simulink model "five_bar_model"  (R2018a)
settings: Solver=ode4  StartTime=0.0  StopTime=10  FixedStep=0.0001  RelTol=1e-3
values from neighbouring files (symbols this model uses):
  g = 9.80665    [ddyn5.m]    (also in idyn5.m = -9.80665; test_dynamics.m = -9.80665; test_model.m)
  q = [NaN; NaN; NaN; NaN; NaN]    [fkine5.m]    (also in ikine5.m = [q11;q12;q13;q21;q22])
  qa = [q11;q21]    [ikine5.m]    (also in model_parameters_v_1.m = ones(length(q_(1,:)),1) * 50; test_model.m = [q(1,:);q(4,:)])
  t0r = J * qda    [ffirstkine5.m]    (also in test_dynamics.m = [0;0]; test_kinematics.m = [1;1]; test_model.m = p)
  t0rd = (J * qdda+ at)    [fsecondkine5.m]    (also in test_dynamics.m = [0;0]; test_kinematics.m = [-1;1]; test_model.m = p)
  x0 = p(1,1)    [model_parameters_v_1.m]    (also in test_model.m)
  y0 = p(2,1)    [model_parameters_v_1.m]    (also in test_model.m = p(1,2))
undefined symbols (not defined in the file or in its folder): X, Y, Z
libraries: sm_lib x23, simulink x10, nesl_utility x9, fl_lib x2
(part 1 of 2)
settings Model: Creator=jere  LastModifiedBy=jere

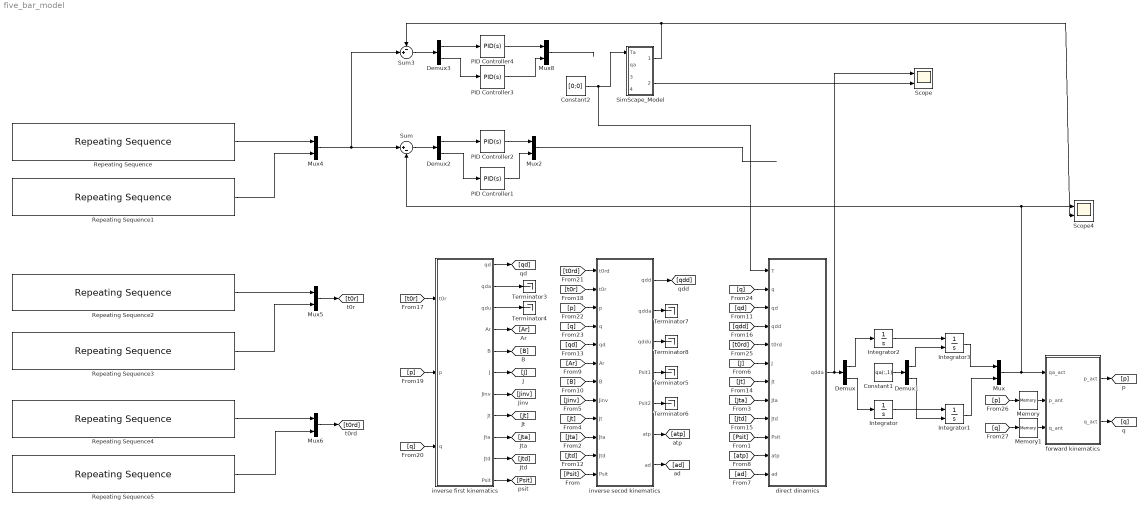
== system five_bar_model ==
  Constant1 : Constant  Value=qa(:,1)
  Constant2 : Constant  Value=[0;0]
  Demux{,1..3} (4 alike) : Demux  Outputs=2
  Integrator : Integrator
  Integrator1 : Integrator  InitialConditionSource=external  InitialCondition=0.3
  Integrator2 : Integrator
  Integrator3 : Integrator  InitialConditionSource=external
  Memory : Memory  InitialCondition=[x0;y0]  LinearizeAsDelay=on
  Memory1 : Memory  InitialCondition=q(:,1)  LinearizeAsDelay=on
  Mux{,2,4..6,8} (6 alike) : Mux  Inputs=2
  PID Controller1 : simulink/Continuous/PID Controller  Controller=PID  TimeDomain=Continuous-time  SampleTime=-1  IntegratorMethod=Forward Euler  FilterMethod=Forward Euler  Form=Parallel  UseFilter=on  ControllerParametersSource=internal  P=75.814948562535  I=487.355305210332  D=2.89544597191695  N=752.857471853223  InitialConditionSource=internal  InitialConditionForIntegrator=0  InitialConditionForFilter=0  ExternalReset=none  LimitOutput=off  UpperSaturationLimit=inf  LowerSaturationLimit=-inf  LinearizeAsGain=on  AntiWindupMode=none  Kb=1  TrackingMode=off  Kt=1  PParamMin=[]  PParamMax=[]  IParamMin=[]  IParamMax=[]  DParamMin=[]  DParamMax=[]  NParamMin=[]  NParamMax=[]  KbParamMin=[]  KbParamMax=[]  KtParamMin=[]  KtParamMax=[]  POutMin=[]  POutMax=[]  IOutMin=[]  IOutMax=[]  DOutMin=[]  DOutMax=[]  NOutMin=[]  NOutMax=[]  KbOutMin=[]  KbOutMax=[]  KtOutMin=[]  KtOutMax=[]  IntegratorOutMin=[]  IntegratorOutMax=[]  FilterOutMin=[]  FilterOutMax=[]  SumOutMin=[]  SumOutMax=[]  SumI1OutMin=[]  SumI1OutMax=[]  SumI2OutMin=[]  SumI2OutMax=[]  SumI3OutMin=[]  SumI3OutMax=[]  SumDOutMin=[]  SumDOutMax=[]  SaturationOutMin=[]  SaturationOutMax=[]  IntegratorContinuousStateAttributes=''  IntegratorStateMustResolveToSignalObject=off  IntegratorRTWStateStorageClass=Auto  FilterContinuousStateAttributes=''  FilterStateMustResolveToSignalObject=off  FilterRTWStateStorageClass=Auto  DifferentiatorICPrevScaledInput=0  DifferentiatorOutMin=[]  DifferentiatorOutMax=[]  FilterDiffOutCoefMin=[]  FilterDiffOutCoefMax=[]  SumDenOutMin=[]  SumDenOutMax=[]  SumNumOutMin=[]  SumNumOutMax=[]  ReciprocalOutMin=[]  ReciprocalOutMax=[]  DivideOutMin=[]  DivideOutMax=[]  TunerSelectOption=Transfer Function Based (PID Tuner App)
  PID Controller2 : simulink/Continuous/PID Controller  Controller=PID  TimeDomain=Continuous-time  SampleTime=-1  IntegratorMethod=Forward Euler  FilterMethod=Forward Euler  Form=Parallel  UseFilter=on  ControllerParametersSource=internal  P=103.663662761202  I=690.778716841285  D=2.91858268707005  N=267.25895733266  InitialConditionSource=internal  InitialConditionForIntegrator=0  InitialConditionForFilter=0  ExternalReset=none  LimitOutput=off  UpperSaturationLimit=inf  LowerSaturationLimit=-inf  LinearizeAsGain=on  AntiWindupMode=none  Kb=1  TrackingMode=off  Kt=1  PParamMin=[]  PParamMax=[]  IParamMin=[]  IParamMax=[]  DParamMin=[]  DParamMax=[]  NParamMin=[]  NParamMax=[]  KbParamMin=[]  KbParamMax=[]  KtParamMin=[]  KtParamMax=[]  POutMin=[]  POutMax=[]  IOutMin=[]  IOutMax=[]  DOutMin=[]  DOutMax=[]  NOutMin=[]  NOutMax=[]  KbOutMin=[]  KbOutMax=[]  KtOutMin=[]  KtOutMax=[]  IntegratorOutMin=[]  IntegratorOutMax=[]  FilterOutMin=[]  FilterOutMax=[]  SumOutMin=[]  SumOutMax=[]  SumI1OutMin=[]  SumI1OutMax=[]  SumI2OutMin=[]  SumI2OutMax=[]  SumI3OutMin=[]  SumI3OutMax=[]  SumDOutMin=[]  SumDOutMax=[]  SaturationOutMin=[]  SaturationOutMax=[]  IntegratorContinuousStateAttributes=''  IntegratorStateMustResolveToSignalObject=off  IntegratorRTWStateStorageClass=Auto  FilterContinuousStateAttributes=''  FilterStateMustResolveToSignalObject=off  FilterRTWStateStorageClass=Auto  DifferentiatorICPrevScaledInput=0  DifferentiatorOutMin=[]  DifferentiatorOutMax=[]  FilterDiffOutCoefMin=[]  FilterDiffOutCoefMax=[]  SumDenOutMin=[]  SumDenOutMax=[]  SumNumOutMin=[]  SumNumOutMax=[]  ReciprocalOutMin=[]  ReciprocalOutMax=[]  DivideOutMin=[]  DivideOutMax=[]  TunerSelectOption=Transfer Function Based (PID Tuner App)
  PID Controller3 : simulink/Continuous/PID Controller  Controller=PID  TimeDomain=Continuous-time  SampleTime=-1  IntegratorMethod=Forward Euler  FilterMethod=Forward Euler  Form=Parallel  UseFilter=on  ControllerParametersSource=internal  P=20220.2005625298  I=4298019.75181635  D=23.0115612854985  N=21654.4579542696  InitialConditionSource=internal  InitialConditionForIntegrator=0  InitialConditionForFilter=0  ExternalReset=none  LimitOutput=off  UpperSaturationLimit=inf  LowerSaturationLimit=-inf  LinearizeAsGain=on  AntiWindupMode=none  Kb=1  TrackingMode=off  Kt=1  PParamMin=[]  PParamMax=[]  IParamMin=[]  IParamMax=[]  DParamMin=[]  DParamMax=[]  NParamMin=[]  NParamMax=[]  KbParamMin=[]  KbParamMax=[]  KtParamMin=[]  KtParamMax=[]  POutMin=[]  POutMax=[]  IOutMin=[]  IOutMax=[]  DOutMin=[]  DOutMax=[]  NOutMin=[]  NOutMax=[]  KbOutMin=[]  KbOutMax=[]  KtOutMin=[]  KtOutMax=[]  IntegratorOutMin=[]  IntegratorOutMax=[]  FilterOutMin=[]  FilterOutMax=[]  SumOutMin=[]  SumOutMax=[]  SumI1OutMin=[]  SumI1OutMax=[]  SumI2OutMin=[]  SumI2OutMax=[]  SumI3OutMin=[]  SumI3OutMax=[]  SumDOutMin=[]  SumDOutMax=[]  SaturationOutMin=[]  SaturationOutMax=[]  IntegratorContinuousStateAttributes=''  IntegratorStateMustResolveToSignalObject=off  IntegratorRTWStateStorageClass=Auto  FilterContinuousStateAttributes=''  FilterStateMustResolveToSignalObject=off  FilterRTWStateStorageClass=Auto  DifferentiatorICPrevScaledInput=0  DifferentiatorOutMin=[]  DifferentiatorOutMax=[]  FilterDiffOutCoefMin=[]  FilterDiffOutCoefMax=[]  SumDenOutMin=[]  SumDenOutMax=[]  SumNumOutMin=[]  SumNumOutMax=[]  ReciprocalOutMin=[]  ReciprocalOutMax=[]  DivideOutMin=[]  DivideOutMax=[]  TunerSelectOption=Transfer Function Based (PID Tuner App)
  PID Controller4 : simulink/Continuous/PID Controller  Controller=PID  TimeDomain=Continuous-time  SampleTime=-1  IntegratorMethod=Forward Euler  FilterMethod=Forward Euler  Form=Parallel  UseFilter=on  ControllerParametersSource=internal  P=130671.244254794  I=70606761.3892061  D=48.6694021998481  N=21806.6233739507  InitialConditionSource=internal  InitialConditionForIntegrator=0  InitialConditionForFilter=0  ExternalReset=none  LimitOutput=off  UpperSaturationLimit=inf  LowerSaturationLimit=-inf  LinearizeAsGain=on  AntiWindupMode=none  Kb=1  TrackingMode=off  Kt=1  PParamMin=[]  PParamMax=[]  IParamMin=[]  IParamMax=[]  DParamMin=[]  DParamMax=[]  NParamMin=[]  NParamMax=[]  KbParamMin=[]  KbParamMax=[]  KtParamMin=[]  KtParamMax=[]  POutMin=[]  POutMax=[]  IOutMin=[]  IOutMax=[]  DOutMin=[]  DOutMax=[]  NOutMin=[]  NOutMax=[]  KbOutMin=[]  KbOutMax=[]  KtOutMin=[]  KtOutMax=[]  IntegratorOutMin=[]  IntegratorOutMax=[]  FilterOutMin=[]  FilterOutMax=[]  SumOutMin=[]  SumOutMax=[]  SumI1OutMin=[]  SumI1OutMax=[]  SumI2OutMin=[]  SumI2OutMax=[]  SumI3OutMin=[]  SumI3OutMax=[]  SumDOutMin=[]  SumDOutMax=[]  SaturationOutMin=[]  SaturationOutMax=[]  IntegratorContinuousStateAttributes=''  IntegratorStateMustResolveToSignalObject=off  IntegratorRTWStateStorageClass=Auto  FilterContinuousStateAttributes=''  FilterStateMustResolveToSignalObject=off  FilterRTWStateStorageClass=Auto  DifferentiatorICPrevScaledInput=0  DifferentiatorOutMin=[]  DifferentiatorOutMax=[]  FilterDiffOutCoefMin=[]  FilterDiffOutCoefMax=[]  SumDenOutMin=[]  SumDenOutMax=[]  SumNumOutMin=[]  SumNumOutMax=[]  ReciprocalOutMin=[]  ReciprocalOutMax=[]  DivideOutMin=[]  DivideOutMax=[]  TunerSelectOption=Transfer Function Based (PID Tuner App)
  Repeating Sequence : simulink/Sources/Repeating Sequence  rep_seq_t=0:10/49:10  rep_seq_y=qa(1,:)
  Repeating Sequence1 : simulink/Sources/Repeating Sequence  rep_seq_t=0:10/49:10  rep_seq_y=qa(2,:)
  Repeating Sequence2 : simulink/Sources/Repeating Sequence  rep_seq_t=0:10/49:10  rep_seq_y=t0r(:,1)'
  Repeating Sequence3 : simulink/Sources/Repeating Sequence  rep_seq_t=0:10/49:10  rep_seq_y=t0r(:,1)'
  Repeating Sequence4 : simulink/Sources/Repeating Sequence  rep_seq_t=0:10/49:10  rep_seq_y=t0rd(:,1)'
  Repeating Sequence5 : simulink/Sources/Repeating Sequence  rep_seq_t=0:10/49:10  rep_seq_y=t0rd(:,2)'
  Scope : Scope  NumInputPorts=2
  Scope4 : Scope  NumInputPorts=2
  SimScape_Model : Subsystem
  Sum : Sum  Inputs=|+-
  Sum3 : Sum  Inputs=-+|
  Terminator{3..8} (6 alike) : Terminator
  direct dinamics : MATLAB Function  TreatAsAtomicUnit=on
  forward kinematics : MATLAB Function  TreatAsAtomicUnit=on
  inverse first kinematics : MATLAB Function  TreatAsAtomicUnit=on
  inverse secod kinematics : MATLAB Function  TreatAsAtomicUnit=on
  wires:
  Integrator/1 -> Integrator1/1
  Integrator2/1 -> Integrator3/1
  Demux/1 -> Integrator2/1
  Demux/2 -> Integrator/1
  Integrator3/1 -> Mux/1
  Integrator1/1 -> Mux/2
  Demux1/1 -> Integrator3/2
  Demux1/2 -> Integrator1/2
  Demux2/2 -> PID Controller1/1
  PID Controller1/1 -> Mux2/2
  direct dinamics/1(qdda) -> Scope/1, Demux/1
  Mux/1 -> Sum/2, Scope4/1, forward kinematics/1(qa_act)
  Repeating Sequence/1 -> Mux4/1
  Repeating Sequence1/1 -> Mux4/2
  Repeating Sequence2/1 -> Mux5/1
  Repeating Sequence3/1 -> Mux5/2
  Repeating Sequence5/1 -> Mux6/2
  Repeating Sequence4/1 -> Mux6/1
  Constant1/1 -> Demux1/1
  Mux4/1 -> Sum/1, Sum3/2
  Demux2/1 -> PID Controller2/1
  inverse first kinematics/2(qda) -> Terminator3/1
  inverse first kinematics/3(qdu) -> Terminator4/1
  Demux3/2 -> PID Controller3/1
  Demux3/1 -> PID Controller4/1
  Sum/1 -> Demux2/1
  Sum3/1 -> Demux3/1
  PID Controller4/1 -> Mux8/1
  PID Controller3/1 -> Mux8/2
  PID Controller2/1 -> Mux2/1
  inverse secod kinematics/4(Psit1) -> Terminator5/1
  inverse secod kinematics/5(Psit2) -> Terminator6/1
  inverse secod kinematics/2(qdda) -> Terminator7/1
  inverse secod kinematics/3(qddu) -> Terminator8/1
  inverse first kinematics/11(Psit) -> [Psit]
  [Psit] -> inverse secod kinematics/12(Psit)
  [Psit] -> direct dinamics/10(Psit)
  inverse first kinematics/9(Jta) -> [Jta]
  [Jta] -> inverse secod kinematics/10(Jta)
  [Jta] -> direct dinamics/8(Jta)
  inverse first kinematics/10(Jtd) -> [Jtd]
  inverse first kinematics/8(Jt) -> [Jt]
  inverse first kinematics/7(Jinv) -> [Jinv]
  inverse first kinematics/6(J) -> [J]
  inverse first kinematics/5(B) -> [B]
  inverse first kinematics/4(Ar) -> [Ar]
  inverse first kinematics/1(qd) -> [qd]
  [Jt] -> inverse secod kinematics/9(Jt)
  [Jinv] -> inverse secod kinematics/8(Jinv)
  [J] -> direct dinamics/6(J)
  inverse secod kinematics/7(ad) -> [ad]
  inverse secod kinematics/6(atp) -> [atp]
  [ad] -> direct dinamics/12(ad)
  [atp] -> direct dinamics/11(atp)
  [Ar] -> inverse secod kinematics/6(Ar)
  [B] -> inverse secod kinematics/7(B)
  [qd] -> direct dinamics/3(qd)
  [Jtd] -> inverse secod kinematics/11(Jtd)
  [qd] -> inverse secod kinematics/5(qd)
  [Jt] -> direct dinamics/7(Jt)
  [Jtd] -> direct dinamics/9(Jtd)
  inverse secod kinematics/1(qdd) -> [qdd]
  [qdd] -> direct dinamics/4(qdd)
  Mux5/1 -> [t0r]
  [t0r] -> inverse first kinematics/1(t0r)
  [t0r] -> inverse secod kinematics/2(t0r)
  forward kinematics/1(p_act) -> [p]
  forward kinematics/2(q_act) -> [q]
  [p] -> inverse first kinematics/2(p)
  [q] -> inverse first kinematics/3(q)
  Mux6/1 -> [t0rd]
  [t0rd] -> inverse secod kinematics/1(t0rd)
  [p] -> inverse secod kinematics/3(p)
  [q] -> inverse secod kinematics/4(q)
  [q] -> direct dinamics/2(q)
  [t0rd] -> direct dinamics/5(t0rd)
  Mux2/1 -> ?
  Mux8/1 -> ?
  SimScape_Model/1(qa_o) -> Scope4/2, Sum3/1
  SimScape_Model/2(qdda_o) -> Scope/2
  [p] -> Memory/1
  Memory/1 -> forward kinematics/2(p_ant)
  Memory1/1 -> forward kinematics/3(q_ant)
  [q] -> Memory1/1
  Constant2/1 -> direct dinamics/1(T), SimScape_Model/1(Ta)

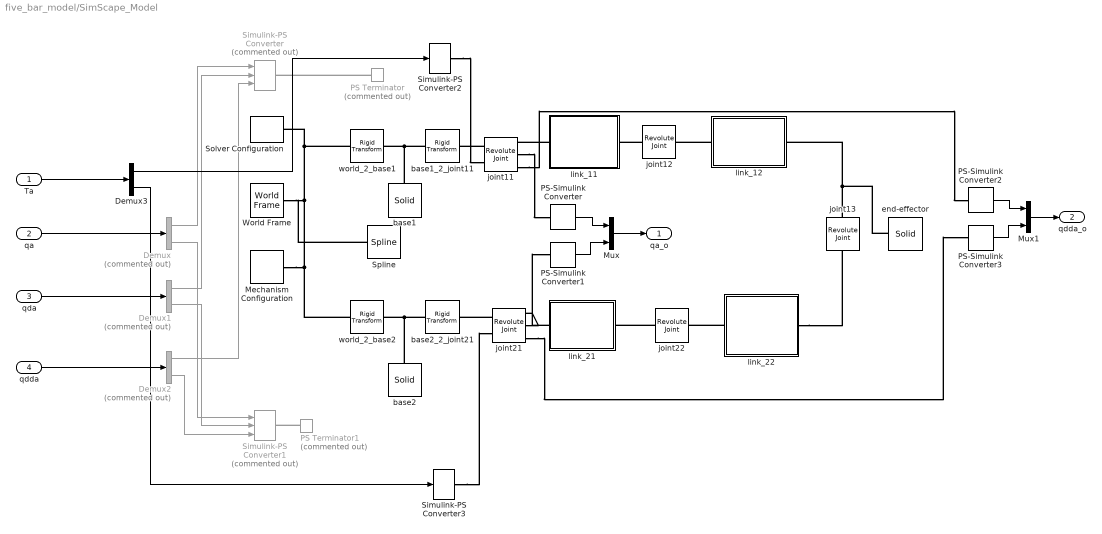
== system five_bar_model/SimScape_Model ==
  Ta : Inport
  qa : Inport  Port=2
  qda : Inport  Port=3
  qdda : Inport  Port=4
  Demux : Demux  Commented=on  Outputs=2
  Demux1 : Demux  Commented=on  Outputs=2
  Demux2 : Demux  Commented=on  Outputs=2
  Demux3 : Demux  Outputs=2
  Mechanism Configuration : sm_lib/Utilities/Mechanism Configuration  UniformGravity=Constant  GravityVector=[0 0 -9.80665]  GravityUnits=m/s^2  LinearizationDelta=0.001
  Mux : Mux  Inputs=2
  Mux1 : Mux  Inputs=2
  PS Terminator : fl_lib/Physical Signals/Sinks/PS Terminator  Commented=on
      settings: SourceProductName=Simscape
  PS Terminator1 : fl_lib/Physical Signals/Sinks/PS Terminator  Commented=on
      settings: SourceProductName=Simscape
  PS-Simulink Converter : nesl_utility/PS-Simulink Converter  PhysicalDomain=network_engine_domain  SubClassName=ps_output  LeftPortType=input  RightPortType=output  PseudoPeriodic=off  Frequencies=[]  Unit=rad  AffineConversion=off
  PS-Simulink Converter1 : nesl_utility/PS-Simulink Converter  PhysicalDomain=network_engine_domain  SubClassName=ps_output  LeftPortType=input  RightPortType=output  PseudoPeriodic=off  Frequencies=[]  Unit=rad  AffineConversion=off
  PS-Simulink Converter2 : nesl_utility/PS-Simulink Converter  PhysicalDomain=network_engine_domain  SubClassName=ps_output  LeftPortType=input  RightPortType=output  PseudoPeriodic=off  Frequencies=[]  Unit=1  AffineConversion=off
  PS-Simulink Converter3 : nesl_utility/PS-Simulink Converter  PhysicalDomain=network_engine_domain  SubClassName=ps_output  LeftPortType=input  RightPortType=output  PseudoPeriodic=off  Frequencies=[]  Unit=1  AffineConversion=off
  Simulink-PS Converter : nesl_utility/Simulink-PS Converter  Commented=on  PhysicalDomain=network_engine_domain  SubClassName=ps_input  LeftPortType=input  RightPortType=output  PseudoPeriodic=off  Frequencies=[]  NoiseDistribution=none  NoiseParameters=[]  Unit=rad  AffineConversion=off  FilteringAndDerivatives=provide  SimscapeFilterOrder=1  InputFilterTimeConstant=0.001  UdotUserProvided=2
  Simulink-PS Converter1 : nesl_utility/Simulink-PS Converter  Commented=on  PhysicalDomain=network_engine_domain  SubClassName=ps_input  LeftPortType=input  RightPortType=output  PseudoPeriodic=off  Frequencies=[]  NoiseDistribution=none  NoiseParameters=[]  Unit=rad  AffineConversion=off  FilteringAndDerivatives=provide  SimscapeFilterOrder=1  InputFilterTimeConstant=0.001  UdotUserProvided=2
  Simulink-PS Converter2 : nesl_utility/Simulink-PS Converter  PhysicalDomain=network_engine_domain  SubClassName=ps_input  LeftPortType=input  RightPortType=output  PseudoPeriodic=off  Frequencies=[]  NoiseDistribution=none  NoiseParameters=[]  Unit=N*m  AffineConversion=off  FilteringAndDerivatives=provide  SimscapeFilterOrder=1  InputFilterTimeConstant=0.001  UdotUserProvided=0
  Simulink-PS Converter3 : nesl_utility/Simulink-PS Converter  PhysicalDomain=network_engine_domain  SubClassName=ps_input  LeftPortType=input  RightPortType=output  PseudoPeriodic=off  Frequencies=[]  NoiseDistribution=none  NoiseParameters=[]  Unit=N*m  AffineConversion=off  FilteringAndDerivatives=provide  SimscapeFilterOrder=1  InputFilterTimeConstant=0.001  UdotUserProvided=0
  Solver Configuration : nesl_utility/Solver Configuration  PhysicalDomain=network_engine_domain  SubClassName=solver  LeftPortType=input  RightPortType=generic  Tones=[]  Harmonics=[]  SimulateNoise=off  Profile=off  UseLocalSampling=off  EnableSwitchedLinearOptims=on  FrequencyDomain=off  UseCCode=off  RelTol=0.001  AbsTol=1e-06  MinStep=1e-09  ToWorkspace=off  RevertToSquareIcSolve=off  NumHomotopyIterations=100  PhasorMode=off  PhasorModeNumHarmonics=1  DoDC=off  ResidualTolerance=1e-09  UseLocalSolver=off  LocalSolverChoice=NE_BACKWARD_EULER_ADVANCER  LocalSolverSampleTime=0.001  DoFixedCost=off  MaxNonlinIter=3  MaxModeIter=2  LinearAlgebra=Sparse  EquationFormulation=NE_TIME_EF  DelaysMemoryBudget=1024  AutomaticFiltering=on  FilteringTimeConstant=0.001
  Spline : sm_lib/Curves and Surfaces/Spline  DataPoints=[-0.1 0.3; 0.1 0.3]  DataPointsUnits=m  EndConditionType=Natural  GraphicType=FromGeometry  MarkerShape=Sphere  MarkerSize=10  GraphicVisPropType=SimpleVisualProperties  GraphicDiffuseColor=[0 0 0]  GraphicSpecularColor=[0.5 0.5 0.5 1.0]  GraphicAmbientColor=[0.15 0.15 0.15 1.0]  GraphicEmissiveColor=[0.0 0.0 0.0 1.0]  GraphicShininess=75  GraphicOpacity=1.0
      settings: SourceProductName=Simscape Multibody
  World Frame : sm_lib/Frames and Transforms/World Frame
  base1 : sm_lib/Body Elements/Solid  InertiaType=PointMass  Mass=1.72  MassUnits=kg  CenterOfMass=[0 0 0]  CenterOfMassUnits=m  MomentsOfInertia=[1 1 1]  MomentsOfInertiaUnits=kg*m^2  ProductsOfInertia=[0 0 0]  ProductsOfInertiaUnits=kg*m^2  DensityBased=on  Density=1000  DensityUnits=kg/m^3  DoExposeReferenceFrame=on  SerializedFrames=<Frames/>  GraphicType=FromGeometry  MarkerShape=Sphere  MarkerSize=10  GraphicVisPropType=SimpleVisualProperties  GraphicDiffuseColor=[1.0 1.0 0.0]  GraphicSpecularColor=[0.5 0.5 0.5 1.0]  GraphicAmbientColor=[0.15 0.15 0.15 1.0]  GraphicEmissiveColor=[0.0 0.0 0.0 1.0]  GraphicShininess=75  GraphicOpacity=1.0  GeometryShape=FromFile  RectangleSize=[1 1]  RectangleSizeUnits=m  BrickDimensions=[1 1 1]  BrickDimensionUnits=m  CylinderRadius=1  CylinderRadiusUnits=m  CylinderLength=1  CylinderLengthUnits=m  SphereRadius=1  SphereRadiusUnits=m  EllipsoidRadii=[1 1 1]  EllipsoidRadiiUnits=m  ExtrusionCrossSection=[1 1; -1 1; -1 -1; 1 -1]  ExtrusionCrossSectionUnits=m  ExtrusionLength=1  ExtrusionLengthUnits=m  PolygonNumSides=3  PolygonOuterRadius=1  PolygonOuterRadiusUnits=m  ExtGeomFileType=STL  ExtGeomFileName=/home/jere/Documentos/simulacionPF/5-bar-model/meshes/nema23_75mm_8mm.stl  ExtGeomFileUnits=mm  RevolutionCrossSection=[1 1; 1 -1; 2 -1; 2 1]  RevolutionCrossSectionUnits=m  RevolutionExtent=Full  RevolutionAngle=180  RevolutionAngleUnits=deg
  base1_2_joint11 : sm_lib/Frames and Transforms/Rigid Transform  TranslationMethod=Cartesian  TranslationStandardOffset=0  TranslationLengthUnit=mm  TranslationStandardAxis=+Z  TranslationCartesianOffset=[0 0 2]  TranslationROffset=0  TranslationROffsetUnits=m  TranslationZOffset=0  TranslationZOffsetUnits=m  TranslationThetaOffset=0  TranslationThetaOffsetUnits=deg  RotationMethod=None  RotationAngleUnits=deg  RotationStandardAxis=+Z  RotationAngle=0.0  RotationArbitraryAxis=[0 0 1]  FollAlignAxisA=+X  BaseAlignAxisA=+Y  FollAlignAxisB=+Y  BaseAlignAxisB=+Z  RotationSequenceAxes=FollowerAxes  RotationSequence=XYX  RotationSequenceAngles=[0 0 0]  RotationSequenceAnglesUnits=deg  RotationMatrix=[1 0 0; 0 1 0; 0 0 1]
  base2 : sm_lib/Body Elements/Solid  InertiaType=PointMass  Mass=1.72  MassUnits=kg  CenterOfMass=[0 0 0]  CenterOfMassUnits=m  MomentsOfInertia=[1 1 1]  MomentsOfInertiaUnits=kg*m^2  ProductsOfInertia=[0 0 0]  ProductsOfInertiaUnits=kg*m^2  DensityBased=on  Density=1000  DensityUnits=kg/m^3  DoExposeReferenceFrame=on  SerializedFrames=<Frames/>  GraphicType=FromGeometry  MarkerShape=Sphere  MarkerSize=10  GraphicVisPropType=SimpleVisualProperties  GraphicDiffuseColor=[1.0 1.0 0.0]  GraphicSpecularColor=[0.5 0.5 0.5 1.0]  GraphicAmbientColor=[0.15 0.15 0.15 1.0]  GraphicEmissiveColor=[0.0 0.0 0.0 1.0]  GraphicShininess=75  GraphicOpacity=1.0  GeometryShape=FromFile  RectangleSize=[1 1]  RectangleSizeUnits=m  BrickDimensions=[1 1 1]  BrickDimensionUnits=m  CylinderRadius=1  CylinderRadiusUnits=m  CylinderLength=1  CylinderLengthUnits=m  SphereRadius=1  SphereRadiusUnits=m  EllipsoidRadii=[1 1 1]  EllipsoidRadiiUnits=m  ExtrusionCrossSection=[1 1; -1 1; -1 -1; 1 -1]  ExtrusionCrossSectionUnits=m  ExtrusionLength=1  ExtrusionLengthUnits=m  PolygonNumSides=3  PolygonOuterRadius=1  PolygonOuterRadiusUnits=m  ExtGeomFileType=STL  ExtGeomFileName=/home/jere/Documentos/simulacionPF/5-bar-model/meshes/nema23_75mm_8mm.stl  ExtGeomFileUnits=mm  RevolutionCrossSection=[1 1; 1 -1; 2 -1; 2 1]  RevolutionCrossSectionUnits=m  RevolutionExtent=Full  RevolutionAngle=180  RevolutionAngleUnits=deg
  base2_2_joint21 : sm_lib/Frames and Transforms/Rigid Transform  TranslationMethod=Cartesian  TranslationStandardOffset=0  TranslationLengthUnit=mm  TranslationStandardAxis=+Z  TranslationCartesianOffset=[0 0 2]  TranslationROffset=0  TranslationROffsetUnits=m  TranslationZOffset=0  TranslationZOffsetUnits=m  TranslationThetaOffset=0  TranslationThetaOffsetUnits=deg  RotationMethod=None  RotationAngleUnits=deg  RotationStandardAxis=+Z  RotationAngle=0.0  RotationArbitraryAxis=[0 0 1]  FollAlignAxisA=+X  BaseAlignAxisA=+Y  FollAlignAxisB=+Y  BaseAlignAxisB=+Z  RotationSequenceAxes=FollowerAxes  RotationSequence=XYX  RotationSequenceAngles=[0 0 0]  RotationSequenceAnglesUnits=deg  RotationMatrix=[1 0 0; 0 1 0; 0 0 1]
  end-effector : sm_lib/Body Elements/Solid  InertiaType=PointMass  Mass=0.272  MassUnits=kg  CenterOfMass=[0 0 0]  CenterOfMassUnits=m  MomentsOfInertia=[1 1 1]  MomentsOfInertiaUnits=kg*m^2  ProductsOfInertia=[0 0 0]  ProductsOfInertiaUnits=kg*m^2  DensityBased=on  Density=1000  DensityUnits=kg/m^3  DoExposeReferenceFrame=on  SerializedFrames=<Frames/>  GraphicType=FromGeometry  MarkerShape=Sphere  MarkerSize=10  GraphicVisPropType=SimpleVisualProperties  GraphicDiffuseColor=[1.0 1.0 0.0]  GraphicSpecularColor=[0.5 0.5 0.5 1.0]  GraphicAmbientColor=[0.15 0.15 0.15 1.0]  GraphicEmissiveColor=[0.0 0.0 0.0 1.0]  GraphicShininess=75  GraphicOpacity=1.0  GeometryShape=Sphere  RectangleSize=[1 1]  RectangleSizeUnits=m  BrickDimensions=[1 1 1]  BrickDimensionUnits=m  CylinderRadius=1  CylinderRadiusUnits=m  CylinderLength=1  CylinderLengthUnits=m  SphereRadius=1  SphereRadiusUnits=mm  EllipsoidRadii=[1 1 1]  EllipsoidRadiiUnits=m  ExtrusionCrossSection=[1 1; -1 1; -1 -1; 1 -1]  ExtrusionCrossSectionUnits=m  ExtrusionLength=1  ExtrusionLengthUnits=m  PolygonNumSides=3  PolygonOuterRadius=1  PolygonOuterRadiusUnits=m  ExtGeomFileType=STL  ExtGeomFileName=D:\PartsMechanism\propiedades\nema23_75mm_8mm.stl  ExtGeomFileUnits=mm  RevolutionCrossSection=[1 1; 1 -1; 2 -1; 2 1]  RevolutionCrossSectionUnits=m  RevolutionExtent=Full  RevolutionAngle=180  RevolutionAngleUnits=deg
  joint11 : sm_lib/Joints/Revolute Joint  SenseConstraintForce=off  SenseConstraintForceX=off  SenseConstraintForceY=off  SenseConstraintForceZ=off  SenseConstraintTorque=off  SenseConstraintTorqueX=off  SenseConstraintTorqueY=off  SenseConstraintTorqueZ=off  SenseTotalForce=off  SenseTotalForceX=off  SenseTotalForceY=off  SenseTotalForceZ=off  SenseTotalTorque=off  SenseTotalTorqueX=off  SenseTotalTorqueY=off  SenseTotalTorqueZ=off  CompositeWrenchDir=FollowerOnBase  CompositeWrenchFrame=BaseFrame  EquilibriumPosition=0  EquilibriumPositionUnits=rad  SpringStiffness=0  SpringStiffnessUnits=N*m/deg  DampingCoefficient=1.5e-5  DampingCoefficientUnits=N*m/(rad/s)  TorqueActuationMode=InputTorque  MotionActuationMode=ComputedMotion  SensePosition=on  SenseVelocity=off  SenseAcceleration=on  SenseTorqueForce=off  PositionTargetSpecify=on  PositionTargetPriority=High  PositionTargetValue=q(1,1)  PositionTargetValueUnits=rad  VelocityTargetSpecify=off  VelocityTargetPriority=High  VelocityTargetValue=1  VelocityTargetValueUnits=rad/s
  joint12 : sm_lib/Joints/Revolute Joint  SenseConstraintForce=off  SenseConstraintForceX=off  SenseConstraintForceY=off  SenseConstraintForceZ=off  SenseConstraintTorque=off  SenseConstraintTorqueX=off  SenseConstraintTorqueY=off  SenseConstraintTorqueZ=off  SenseTotalForce=off  SenseTotalForceX=off  SenseTotalForceY=off  SenseTotalForceZ=off  SenseTotalTorque=off  SenseTotalTorqueX=off  SenseTotalTorqueY=off  SenseTotalTorqueZ=off  CompositeWrenchDir=FollowerOnBase  CompositeWrenchFrame=BaseFrame  EquilibriumPosition=0  EquilibriumPositionUnits=rad  SpringStiffness=0  SpringStiffnessUnits=N*m/deg  DampingCoefficient=0  DampingCoefficientUnits=N*m/(rad/s)  TorqueActuationMode=NoTorque  MotionActuationMode=ComputedMotion  SensePosition=off  SenseVelocity=off  SenseAcceleration=off  SenseTorqueForce=off  PositionTargetSpecify=off  PositionTargetPriority=High  PositionTargetValue=q(2,1)  PositionTargetValueUnits=rad  VelocityTargetSpecify=off  VelocityTargetPriority=High  VelocityTargetValue=100  VelocityTargetValueUnits=rad/s
  joint13 : sm_lib/Joints/Revolute Joint  SenseConstraintForce=off  SenseConstraintForceX=off  SenseConstraintForceY=off  SenseConstraintForceZ=off  SenseConstraintTorque=off  SenseConstraintTorqueX=off  SenseConstraintTorqueY=off  SenseConstraintTorqueZ=off  SenseTotalForce=off  SenseTotalForceX=off  SenseTotalForceY=off  SenseTotalForceZ=off  SenseTotalTorque=off  SenseTotalTorqueX=off  SenseTotalTorqueY=off  SenseTotalTorqueZ=off  CompositeWrenchDir=FollowerOnBase  CompositeWrenchFrame=BaseFrame  EquilibriumPosition=0  EquilibriumPositionUnits=rad  SpringStiffness=0  SpringStiffnessUnits=N*m/deg  DampingCoefficient=0  DampingCoefficientUnits=N*m/(rad/s)  TorqueActuationMode=NoTorque  MotionActuationMode=ComputedMotion  SensePosition=off  SenseVelocity=off  SenseAcceleration=off  SenseTorqueForce=off  PositionTargetSpecify=off  PositionTargetPriority=High  PositionTargetValue=270  PositionTargetValueUnits=rad  VelocityTargetSpecify=off  VelocityTargetPriority=High  VelocityTargetValue=100  VelocityTargetValueUnits=rad/s
  joint21 : sm_lib/Joints/Revolute Joint  SenseConstraintForce=off  SenseConstraintForceX=off  SenseConstraintForceY=off  SenseConstraintForceZ=off  SenseConstraintTorque=off  SenseConstraintTorqueX=off  SenseConstraintTorqueY=off  SenseConstraintTorqueZ=off  SenseTotalForce=off  SenseTotalForceX=off  SenseTotalForceY=off  SenseTotalForceZ=off  SenseTotalTorque=off  SenseTotalTorqueX=off  SenseTotalTorqueY=off  SenseTotalTorqueZ=off  CompositeWrenchDir=FollowerOnBase  CompositeWrenchFrame=BaseFrame  EquilibriumPosition=0  EquilibriumPositionUnits=rad  SpringStiffness=0  SpringStiffnessUnits=N*m/deg  DampingCoefficient=1.5e-5  DampingCoefficientUnits=N*m/(rad/s)  TorqueActuationMode=InputTorque  MotionActuationMode=ComputedMotion  SensePosition=on  SenseVelocity=off  SenseAcceleration=on  SenseTorqueForce=off  PositionTargetSpecify=on  PositionTargetPriority=High  PositionTargetValue=q(4,1)  PositionTargetValueUnits=rad  VelocityTargetSpecify=off  VelocityTargetPriority=High  VelocityTargetValue=100  VelocityTargetValueUnits=rad/s
  joint22 : sm_lib/Joints/Revolute Joint  SenseConstraintForce=off  SenseConstraintForceX=off  SenseConstraintForceY=off  SenseConstraintForceZ=off  SenseConstraintTorque=off  SenseConstraintTorqueX=off  SenseConstraintTorqueY=off  SenseConstraintTorqueZ=off  SenseTotalForce=off  SenseTotalForceX=off  SenseTotalForceY=off  SenseTotalForceZ=off  SenseTotalTorque=off  SenseTotalTorqueX=off  SenseTotalTorqueY=off  SenseTotalTorqueZ=off  CompositeWrenchDir=FollowerOnBase  CompositeWrenchFrame=BaseFrame  EquilibriumPosition=0  EquilibriumPositionUnits=rad  SpringStiffness=0  SpringStiffnessUnits=N*m/deg  DampingCoefficient=0  DampingCoefficientUnits=N*m/(rad/s)  TorqueActuationMode=NoTorque  MotionActuationMode=ComputedMotion  SensePosition=off  SenseVelocity=off  SenseAcceleration=off  SenseTorqueForce=off  PositionTargetSpecify=off  PositionTargetPriority=High  PositionTargetValue=q(5,1)  PositionTargetValueUnits=rad  VelocityTargetSpecify=off  VelocityTargetPriority=High  VelocityTargetValue=100  VelocityTargetValueUnits=rad/s
  link_11 : Subsystem
  link_12 : Subsystem
  link_21 : Subsystem
  link_22 : Subsystem
  world_2_base1 : sm_lib/Frames and Transforms/Rigid Transform  TranslationMethod=Cartesian  TranslationStandardOffset=0  TranslationLengthUnit=mm  TranslationStandardAxis=+Z  TranslationCartesianOffset=[-125 0 0]  TranslationROffset=0  TranslationROffsetUnits=m  TranslationZOffset=0  TranslationZOffsetUnits=m  TranslationThetaOffset=0  TranslationThetaOffsetUnits=deg  RotationMethod=None  RotationAngleUnits=deg  RotationStandardAxis=+Z  RotationAngle=0.0  RotationArbitraryAxis=[0 0 1]  FollAlignAxisA=+X  BaseAlignAxisA=+Y  FollAlignAxisB=+Y  BaseAlignAxisB=+Z  RotationSequenceAxes=FollowerAxes  RotationSequence=XYX  RotationSequenceAngles=[0 0 0]  RotationSequenceAnglesUnits=deg  RotationMatrix=[1 0 0; 0 1 0; 0 0 1]
  world_2_base2 : sm_lib/Frames and Transforms/Rigid Transform  TranslationMethod=Cartesian  TranslationStandardOffset=0  TranslationLengthUnit=mm  TranslationStandardAxis=+Z  TranslationCartesianOffset=[125 0 0]  TranslationROffset=0  TranslationROffsetUnits=m  TranslationZOffset=0  TranslationZOffsetUnits=m  TranslationThetaOffset=0  TranslationThetaOffsetUnits=deg  RotationMethod=None  RotationAngleUnits=deg  RotationStandardAxis=+Z  RotationAngle=0.0  RotationArbitraryAxis=[0 0 1]  FollAlignAxisA=+X  BaseAlignAxisA=+Y  FollAlignAxisB=+Y  BaseAlignAxisB=+Z  RotationSequenceAxes=FollowerAxes  RotationSequence=XYX  RotationSequenceAngles=[0 0 0]  RotationSequenceAnglesUnits=deg  RotationMatrix=[1 0 0; 0 1 0; 0 0 1]
  qa_o : Outport
  qdda_o : Outport  Port=2
  wires:
  PS-Simulink Converter/1 -> Mux/1
  PS-Simulink Converter3/1 -> Mux1/2
  Demux/1 -> Simulink-PS Converter/1
  PS-Simulink Converter1/1 -> Mux/2
  PS-Simulink Converter2/1 -> Mux1/1
  Mux/1 -> qa_o/1
  Demux/2 -> Simulink-PS Converter1/1
  Mux1/1 -> qdda_o/1
  qa/1 -> Demux/1
  Demux1/2 -> Simulink-PS Converter1/2
  Demux1/1 -> Simulink-PS Converter/2
  qda/1 -> Demux1/1
  Demux2/2 -> Simulink-PS Converter1/3
  Demux2/1 -> Simulink-PS Converter/3
  qdda/1 -> Demux2/1
  Ta/1 -> Demux3/1
  Demux3/1 -> Simulink-PS Converter2/1
  Demux3/2 -> Simulink-PS Converter3/1
  connections:
  joint12/LConn1 -- link_11/RConn1
  joint22/LConn1 -- link_21/RConn1
  world_2_base2/LConn1 -- Mechanism Configuration/RConn1 -- Spline/LConn1 -- World Frame/RConn1 -- world_2_base1/LConn1 -- Solver Configuration/RConn1
  link_21/LConn1 -- joint21/RConn1
  base1/RConn1 -- base1_2_joint11/LConn1 -- world_2_base1/RConn1
  base2_2_joint21/LConn1 -- base2/RConn1 -- world_2_base2/RConn1
  joint11/LConn1 -- base1_2_joint11/RConn1
  link_11/LConn1 -- joint11/RConn1
  joint21/LConn1 -- base2_2_joint21/RConn1
  joint13/LConn1 -- end-effector/RConn1 -- link_12/RConn1
  link_22/RConn1 -- joint13/RConn1
  link_22/LConn1 -- joint22/RConn1
  link_12/LConn1 -- joint12/RConn1
  joint11/RConn2 -- PS-Simulink Converter/LConn1
  joint21/RConn2 -- PS-Simulink Converter1/LConn1
  joint21/RConn3 -- PS-Simulink Converter3/LConn1
  joint11/RConn3 -- PS-Simulink Converter2/LConn1
  PS Terminator/LConn1 -- Simulink-PS Converter/RConn1
  PS Terminator1/LConn1 -- Simulink-PS Converter1/RConn1
  Simulink-PS Converter2/RConn1 -- joint11/LConn2
  Simulink-PS Converter3/RConn1 -- joint21/LConn2

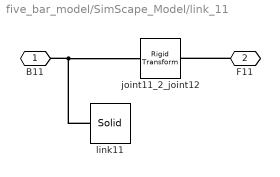
== system five_bar_model/SimScape_Model/link_11 ==
  joint11_2_joint12 : sm_lib/Frames and Transforms/Rigid Transform  TranslationMethod=Cartesian  TranslationStandardOffset=0  TranslationLengthUnit=mm  TranslationStandardAxis=+Z  TranslationCartesianOffset=[205 -3 20]  TranslationROffset=0  TranslationROffsetUnits=m  TranslationZOffset=0  TranslationZOffsetUnits=m  TranslationThetaOffset=0  TranslationThetaOffsetUnits=deg  RotationMethod=None  RotationAngleUnits=deg  RotationStandardAxis=+Z  RotationAngle=0.0  RotationArbitraryAxis=[0 0 1]  FollAlignAxisA=+X  BaseAlignAxisA=+Y  FollAlignAxisB=+Y  BaseAlignAxisB=+Z  RotationSequenceAxes=FollowerAxes  RotationSequence=XYX  RotationSequenceAngles=[0 0 0]  RotationSequenceAnglesUnits=deg  RotationMatrix=[1 0 0; 0 1 0; 0 0 1]
  link11 : sm_lib/Body Elements/Solid  InertiaType=Custom  Mass=83.731  MassUnits=g  CenterOfMass=[1.44 8.82 1.19]  CenterOfMassUnits=cm  MomentsOfInertia=[5653.251 63.763 5693.528]  MomentsOfInertiaUnits=g*cm^2  ProductsOfInertia=[0 0 0]  ProductsOfInertiaUnits=g*cm^2  DensityBased=on  Density=1000  DensityUnits=kg/m^3  DoExposeReferenceFrame=off  SerializedFrames=<Frames><Frame><Id>Frame1</Id><Value><Name>F1</Name><Origin><Source>ReferenceFrame</Source><FeatureName></FeatureName></Origin><PrimaryAxis><DefinedDirection>+Z</DefinedDirection><Source>ReferenceFrame</Source><SourceDirection>+Z</SourceDirection><FeatureName></FeatureName></PrimaryAxis><SecondaryAxis><DefinedDirection>+X</DefinedDirection><Source>ReferenceFrame</Source><SourceDirection>+Y</SourceDirection><FeatureName></FeatureName></SecondaryAxis></Value></Frame></Frames>  GraphicType=FromGeometry  MarkerShape=Sphere  MarkerSize=10  GraphicVisPropType=SimpleVisualProperties  GraphicDiffuseColor=[0.0 0.0 0.8]  GraphicSpecularColor=[0.5 0.5 0.5 1.0]  GraphicAmbientColor=[0.15 0.15 0.15 1.0]  GraphicEmissiveColor=[0.0 0.0 0.0 1.0]  GraphicShininess=75  GraphicOpacity=1.0  GeometryShape=FromFile  RectangleSize=[1 1]  RectangleSizeUnits=m  BrickDimensions=[1 1 1]  BrickDimensionUnits=m  CylinderRadius=1  CylinderRadiusUnits=m  CylinderLength=1  CylinderLengthUnits=m  SphereRadius=1  SphereRadiusUnits=m  EllipsoidRadii=[1 1 1]  EllipsoidRadiiUnits=m  ExtrusionCrossSection=[1 1; -1 1; -1 -1; 1 -1]  ExtrusionCrossSectionUnits=m  ExtrusionLength=1  ExtrusionLengthUnits=m  PolygonNumSides=3  PolygonOuterRadius=1  PolygonOuterRadiusUnits=m  ExtGeomFileType=STL  ExtGeomFileName=/home/jere/Documentos/simulacionPF/5-bar-model/meshes/link_11.stl  ExtGeomFileUnits=mm  RevolutionCrossSection=[1 1; 1 -1; 2 -1; 2 1]  RevolutionCrossSectionUnits=m  RevolutionExtent=Full  RevolutionAngle=180  RevolutionAngleUnits=deg
  B11 : PMIOPort  Side=Left
  F11 : PMIOPort  Port=2  Side=Right
  connections:
  F11/RConn1 -- joint11_2_joint12/RConn1
  link11/LConn1 -- B11/RConn1 -- joint11_2_joint12/LConn1

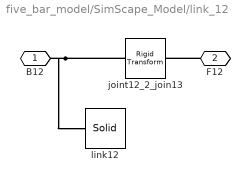
== system five_bar_model/SimScape_Model/link_12 ==
  joint12_2_join13 : sm_lib/Frames and Transforms/Rigid Transform  TranslationMethod=Cartesian  TranslationStandardOffset=0  TranslationLengthUnit=mm  TranslationStandardAxis=+Z  TranslationCartesianOffset=[205 0 15]  TranslationROffset=0  TranslationROffsetUnits=m  TranslationZOffset=0  TranslationZOffsetUnits=m  TranslationThetaOffset=0  TranslationThetaOffsetUnits=deg  RotationMethod=None  RotationAngleUnits=deg  RotationStandardAxis=+Z  RotationAngle=0.0  RotationArbitraryAxis=[0 0 1]  FollAlignAxisA=+X  BaseAlignAxisA=+Y  FollAlignAxisB=+Y  BaseAlignAxisB=+Z  RotationSequenceAxes=FollowerAxes  RotationSequence=XYX  RotationSequenceAngles=[0 0 0]  RotationSequenceAnglesUnits=deg  RotationMatrix=[1 0 0; 0 1 0; 0 0 1]
  link12 : sm_lib/Body Elements/Solid  InertiaType=Custom  Mass=72.020  MassUnits=g  CenterOfMass=[-1.24 10.25 0.75]  CenterOfMassUnits=cm  MomentsOfInertia=[4580.984 35.23 4605.847]  MomentsOfInertiaUnits=g*cm^2  ProductsOfInertia=[0 0 0]  ProductsOfInertiaUnits=g*cm^2  DensityBased=on  Density=1000  DensityUnits=kg/m^3  DoExposeReferenceFrame=off  SerializedFrames=<Frames><Frame><Id>Frame1</Id><Value><Name>F1</Name><Origin><Source>ReferenceFrame</Source><FeatureName></FeatureName></Origin><PrimaryAxis><DefinedDirection>+Z</DefinedDirection><Source>ReferenceFrame</Source><SourceDirection>+Z</SourceDirection><FeatureName></FeatureName></PrimaryAxis><SecondaryAxis><DefinedDirection>+X</DefinedDirection><Source>ReferenceFrame</Source><SourceDirection>+Y</SourceDirection><FeatureName></FeatureName></SecondaryAxis></Value></Frame></Frames>  GraphicType=FromGeometry  MarkerShape=Sphere  MarkerSize=10  GraphicVisPropType=SimpleVisualProperties  GraphicDiffuseColor=[0.0 0.8 0.0]  GraphicSpecularColor=[0.5 0.5 0.5 1.0]  GraphicAmbientColor=[0.15 0.15 0.15 1.0]  GraphicEmissiveColor=[0.0 0.0 0.0 1.0]  GraphicShininess=75  GraphicOpacity=1.0  GeometryShape=FromFile  RectangleSize=[1 1]  RectangleSizeUnits=m  BrickDimensions=[1 1 1]  BrickDimensionUnits=m  CylinderRadius=1  CylinderRadiusUnits=m  CylinderLength=1  CylinderLengthUnits=m  SphereRadius=1  SphereRadiusUnits=m  EllipsoidRadii=[1 1 1]  EllipsoidRadiiUnits=m  ExtrusionCrossSection=[1 1; -1 1; -1 -1; 1 -1]  ExtrusionCrossSectionUnits=m  ExtrusionLength=1  ExtrusionLengthUnits=m  PolygonNumSides=3  PolygonOuterRadius=1  PolygonOuterRadiusUnits=m  ExtGeomFileType=STL  ExtGeomFileName=/home/jere/Documentos/simulacionPF/5-bar-model/meshes/link_12.stl  ExtGeomFileUnits=mm  RevolutionCrossSection=[1 1; 1 -1; 2 -1; 2 1]  RevolutionCrossSectionUnits=m  RevolutionExtent=Full  RevolutionAngle=180  RevolutionAngleUnits=deg
  B12 : PMIOPort  Side=Left
  F12 : PMIOPort  Port=2  Side=Right
  connections:
  F12/RConn1 -- joint12_2_join13/RConn1
  B12/RConn1 -- link12/LConn1 -- joint12_2_join13/LConn1

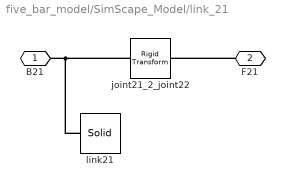
== system five_bar_model/SimScape_Model/link_21 ==
  joint21_2_joint22 : sm_lib/Frames and Transforms/Rigid Transform  TranslationMethod=Cartesian  TranslationStandardOffset=0  TranslationLengthUnit=mm  TranslationStandardAxis=+Z  TranslationCartesianOffset=[205 -31 35]  TranslationROffset=0  TranslationROffsetUnits=m  TranslationZOffset=0  TranslationZOffsetUnits=m  TranslationThetaOffset=0  TranslationThetaOffsetUnits=deg  RotationMethod=None  RotationAngleUnits=deg  RotationStandardAxis=+Z  RotationAngle=0  RotationArbitraryAxis=[0 0 1]  FollAlignAxisA=+X  BaseAlignAxisA=+Y  FollAlignAxisB=+Y  BaseAlignAxisB=+Z  RotationSequenceAxes=FollowerAxes  RotationSequence=XYX  RotationSequenceAngles=[0 0 0]  RotationSequenceAnglesUnits=deg  RotationMatrix=[1 0 0; 0 1 0; 0 0 1]
  link21 : sm_lib/Body Elements/Solid  InertiaType=Custom  Mass=102.422  MassUnits=g  CenterOfMass=[1.48 7.21 2.33]  CenterOfMassUnits=cm  MomentsOfInertia=[6910.383 160.537 6923.992]  MomentsOfInertiaUnits=g*cm^2  ProductsOfInertia=[329.041 20.475 275.874]  ProductsOfInertiaUnits=g*cm^2  DensityBased=on  Density=1000  DensityUnits=kg/m^3  DoExposeReferenceFrame=off  SerializedFrames=<Frames><Frame><Id>Frame1</Id><Value><Name>F1</Name><Origin><Source>ReferenceFrame</Source><FeatureName></FeatureName></Origin><PrimaryAxis><DefinedDirection>+Z</DefinedDirection><Source>ReferenceFrame</Source><SourceDirection>+Z</SourceDirection><FeatureName></FeatureName></PrimaryAxis><SecondaryAxis><DefinedDirection>+X</DefinedDirection><Source>ReferenceFrame</Source><SourceDirection>+Y</SourceDirection><FeatureName></FeatureName></SecondaryAxis></Value></Frame></Frames>  GraphicType=FromGeometry  MarkerShape=Sphere  MarkerSize=10  GraphicVisPropType=SimpleVisualProperties  GraphicDiffuseColor=[0.0 0.0 0.8]  GraphicSpecularColor=[0.5 0.5 0.5 1.0]  GraphicAmbientColor=[0.15 0.15 0.15 1.0]  GraphicEmissiveColor=[0.0 0.0 0.0 1.0]  GraphicShininess=75  GraphicOpacity=1.0  GeometryShape=FromFile  RectangleSize=[1 1]  RectangleSizeUnits=m  BrickDimensions=[1 1 1]  BrickDimensionUnits=m  CylinderRadius=1  CylinderRadiusUnits=m  CylinderLength=1  CylinderLengthUnits=m  SphereRadius=1  SphereRadiusUnits=m  EllipsoidRadii=[1 1 1]  EllipsoidRadiiUnits=m  ExtrusionCrossSection=[1 1; -1 1; -1 -1; 1 -1]  ExtrusionCrossSectionUnits=m  ExtrusionLength=1  ExtrusionLengthUnits=m  PolygonNumSides=3  PolygonOuterRadius=1  PolygonOuterRadiusUnits=m  ExtGeomFileType=STL  ExtGeomFileName=/home/jere/Documentos/simulacionPF/5-bar-model/meshes/link_21.stl  ExtGeomFileUnits=mm  RevolutionCrossSection=[1 1; 1 -1; 2 -1; 2 1]  RevolutionCrossSectionUnits=m  RevolutionExtent=Full  RevolutionAngle=180  RevolutionAngleUnits=deg
  B21 : PMIOPort  Side=Left
  F21 : PMIOPort  Port=2  Side=Right
  connections:
  F21/RConn1 -- joint21_2_joint22/RConn1
  link21/LConn1 -- joint21_2_joint22/LConn1 -- B21/RConn1

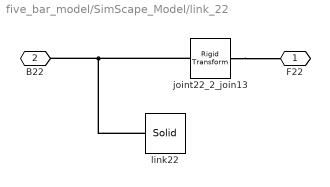
== system five_bar_model/SimScape_Model/link_22 ==
  joint22_2_join13 : sm_lib/Frames and Transforms/Rigid Transform  TranslationMethod=Cartesian  TranslationStandardOffset=0  TranslationLengthUnit=mm  TranslationStandardAxis=+Z  TranslationCartesianOffset="[205 0  0]"  TranslationROffset=0  TranslationROffsetUnits=m  TranslationZOffset=0  TranslationZOffsetUnits=m  TranslationThetaOffset=0  TranslationThetaOffsetUnits=deg  RotationMethod=None  RotationAngleUnits=deg  RotationStandardAxis=+Z  RotationAngle=0.0  RotationArbitraryAxis=[0 0 1]  FollAlignAxisA=+X  BaseAlignAxisA=+Y  FollAlignAxisB=+Y  BaseAlignAxisB=+Z  RotationSequenceAxes=FollowerAxes  RotationSequence=XYX  RotationSequenceAngles=[0 0 0]  RotationSequenceAnglesUnits=deg  RotationMatrix=[1 0 0; 0 1 0; 0 0 1]
  link22 : sm_lib/Body Elements/Solid  InertiaType=Custom  Mass=72.020  MassUnits=g  CenterOfMass=[1.24 10.25 0.75]  CenterOfMassUnits=cm  MomentsOfInertia=[4580.628 35.273 4606.029]  MomentsOfInertiaUnits=g*cm^2  ProductsOfInertia=[0 0 0]  ProductsOfInertiaUnits=g*cm^2  DensityBased=on  Density=1000  DensityUnits=kg/m^3  DoExposeReferenceFrame=off  SerializedFrames=<Frames><Frame><Id>Frame1</Id><Value><Name>F1</Name><Origin><Source>ReferenceFrame</Source><FeatureName></FeatureName></Origin><PrimaryAxis><DefinedDirection>+Z</DefinedDirection><Source>ReferenceFrame</Source><SourceDirection>+Z</SourceDirection><FeatureName></FeatureName></PrimaryAxis><SecondaryAxis><DefinedDirection>+X</DefinedDirection><Source>ReferenceFrame</Source><SourceDirection>+Y</SourceDirection><FeatureName></FeatureName></SecondaryAxis></Value></Frame></Frames>  GraphicType=FromGeometry  MarkerShape=Sphere  MarkerSize=10  GraphicVisPropType=SimpleVisualProperties  GraphicDiffuseColor=[0.0 0.8 0.0]  GraphicSpecularColor=[0.5 0.5 0.5 1.0]  GraphicAmbientColor=[0.15 0.15 0.15 1.0]  GraphicEmissiveColor=[0.0 0.0 0.0 1.0]  GraphicShininess=75  GraphicOpacity=1.0  GeometryShape=FromFile  RectangleSize=[1 1]  RectangleSizeUnits=m  BrickDimensions=[1 1 1]  BrickDimensionUnits=m  CylinderRadius=1  CylinderRadiusUnits=m  CylinderLength=1  CylinderLengthUnits=m  SphereRadius=1  SphereRadiusUnits=m  EllipsoidRadii=[1 1 1]  EllipsoidRadiiUnits=m  ExtrusionCrossSection=[1 1; -1 1; -1 -1; 1 -1]  ExtrusionCrossSectionUnits=m  ExtrusionLength=1  ExtrusionLengthUnits=m  PolygonNumSides=3  PolygonOuterRadius=1  PolygonOuterRadiusUnits=m  ExtGeomFileType=STL  ExtGeomFileName=/home/jere/Documentos/simulacionPF/5-bar-model/meshes/link_22.stl  ExtGeomFileUnits=mm  RevolutionCrossSection=[1 1; 1 -1; 2 -1; 2 1]  RevolutionCrossSectionUnits=m  RevolutionExtent=Full  RevolutionAngle=180  RevolutionAngleUnits=deg
  F22 : PMIOPort  Side=Right
  B22 : PMIOPort  Port=2  Side=Left
  connections:
  joint22_2_join13/RConn1 -- F22/RConn1
  link22/LConn1 -- joint22_2_join13/LConn1 -- B22/RConn1

== matlab function five_bar_model/direct dinamics ==
  data: T input; qdda output size=2; q input; qd input; qdd input; t0rd input; J input; Jt input; Jta input; Jtd input; Psit input; atp input; ad input
function qdda  = ddyn5(T,q,qd,qdd,t0rd,J,Jt,Jta,Jtd,Psit,atp,ad)
% @return qdda: matrix 2x1
    l = 0.205;
    d0 = 0.125;
    d1 = [-d0, l, l];
    d2 = [d0, l, l];
    q1 = q(1:3);
    q2 = q(4:5);
    qd1 = qd(1:3);
    qd2 = qd(4:5);
    qdd1 = qdd(1:3);
    qdd2 = qdd(4:5);
    xdd = t0rd(1);
    ydd = t0rd(2);
    qdda = [0;0];
    % Numerical Solution Dynamic
    m12 = 83.731e-3; %kg
    mx12 = m12 * 8.82e-2;
    my12 = m12 * 1.44e-2;
    m22 = 102.422e-3; %kg
    mx22= m22 * 7.21e-2;
    my22= m22 * 1.48e-2;

    zz12 = 12283.918e-7;
    zz22 = 12283.918e-7;
    %Fricciones fv = viscosa fs= seca
    fv1 = [1.5e-5 0 0];
    fs1 = [1.5e-5 0 0];
    fv2 = [0 0];
    fs2 = [0 0];
    
    zz11 = 12375.675e-7; % kg-m²
    Ia11 = 0.48 * 0.0001; % kg-m2
    zz11r = zz11 + Ia11 + d1(2)^2 * m12;
%     zz11r = 2.11e-2;

    zz21 = 12469.254e-7; % kg-m²
    Ia21 = 0.48 * 0.0001; % kg-m2
    zz21r = zz21 + Ia21 + d2(2)^2 * m22;
%     zz21r = 2.24e-2;
    m4 = 0.272;
    xdd = t0rd(1);
    ydd = t0rd(2);
    % Direct dynamics model
    M11 = zz11r + zz12 + 2 * d1(2) * mx12 * cos(q1(2)) + ...
          2 * d1(2) * my12 * sin(q1(2));

    M12 = zz12 + d1(2) * mx12 * cos(q1(2)) + ...
          d1(2) * my12 * sin(q1(2));
    M21 = M12;

    M44 = zz21r + zz22 + 2 * d2(2) * mx22 * cos(q2(2)) + ...
          2 * d2(2) * my22 * sin(q2(2));

    M45 = zz22 + d2(2) * mx22 * cos(q2(2)) + ...
          d2(2) * my22 * sin(q2(2));
    M54 = M45;

    Mt = [M11 M12  0 0     0;
          M21 zz12 0 0     0;
          0   0    0 0     0;
          0   0    0 M44 M45;
          0   0    0 M54 zz22];

    c1 = -d1(2) * mx12 * qd1(2) * (2 * qd1(1) + qd1(2)) * sin(q1(2)) + ...
         d1(2) * my12 * qd1(2) * (2 * qd1(1) + qd1(2)) * cos(q1(2)) + ...
         fs1(1) * sign(qd1(1)) + fv1(1) * qd1(1);

    c2 = d1(2) * mx12 * qd1(1)^2 * sin(q1(2)) - ...
         d1(2) * my12 * qd1(1)^2 * cos(q1(2)) + ...
         fs1(2) * sign(qd1(2)) + fv1(2) * qd1(2);

    c3 = fs1(3)*sign(qd1(3)) + fv1(3)*qd1(3);

    c4 = -d2(2) * mx22 * qd2(2) * (2 * qd2(1) + qd2(2) ) * sin(q2(2)) + ...
         d2(2) * my22 * qd2(2) * (2 * qd2(1) + qd2(2) ) * cos(q2(2)) + ...
         fs2(1) * sign( qd2(1) ) + fv2(1) * qd2(1);

    c5 = d2(2) * mx22 * qd2(1)^2 * sin(q2(2)) - ...
         d2(2) * my22 * qd2(1)^2 * cos(q2(2)) + ...
         fs2(2) * sign(qd2(2)) + fv2(2) * qd2(2);

    ct = [c1; c2; c3; c4; c5];

    Et = [1 0 0 0 0;
          0 0 1 0 0;
          0 0 0 1 0;
          0 1 0 0 0;
          0 0 0 0 1];

    M0p = m4 * [eye(2), zeros(2,4); zeros(4,2), zeros(4)];
    % c0p = zeros(6,1);
    w0p_ = M0p * [xdd; ydd; zeros(4,1)]; % + c0p;

    % M0r = Psit' * M0p * Psit; % Igual a m4*eye(2)
    M0r = m4 * eye(2);

    Jd = inv(Jtd) * (Jt * J - Jta);

    M = [eye(2), Jd'] * Et'*Mt*Et * [eye(2);Jd] + J'*M0r*J;

        % wr1 = [cos(q1(1)+q1(2)); sin(q1(1)+q1(2)); 0; 0; 0; 0];
        % wr2 = [cos(q2(1)+q2(2)); sin(q2(1)+q2(2)); 0; 0; 0; 0];

        % b0p1 = [-d1(2)*qd1(1)*cos(q1(1)) - d1(3)*cos(q1(1)+q1(2))*(qd1(1)+qd1(2)); -d1(2)*qd1(1)*sin(q1(1)) - d1(3)*sin(q1(1)+q1(2))*(qd1(1)+qd1(2)); 0; 0; 0; 0] * qd1(1) + [- d1(3)*cos(q1(1)+q1(2));- d1(3)*sin(q1(1)+q1(2)); 0; 0; 0; 0] * qd1(2)*(qd1(1)+qd1(2));
        % b0p2 = [-d2(2)*qd2(1)*cos(q2(1)) - d2(3)*cos(q2(1)+q2(2))*(qd2(1)+qd2(2)); -d2(2)*qd2(1)*sin(q2(1)) - d2(3)*sin(q2(1)+q2(2))*(qd2(1)+qd2(2)); 0; 0; 0; 0] * qd2(1) + [- d2(3)*cos(q2(1)+q2(2));- d2(3)*sin(q2(1)+q2(2)); 0; 0; 0; 0] * qd2(2)*(qd2(1)+qd2(2));

        % b0p = [wr1'*b0p1; wr2'*b0p2];
    % b0pr = b0p; % - A * Psidt * t0rn; % Its b0p

    % at_ = -inv(Ar)*b0pr;
    % atp = Psit * at + Psidt * t0rn;
    % atp_ = Psit * at_ + Psidt * t0rn

    c0r = M0p * atp; % Debe ser igual a 0
    % c0r = (M0p * atp_) % Debe ser igual a 0
    % c0r = zeros(6,1);

    % ad = inv(Jtd) * (dc + Jt*at);
    % ad_ = inv(Jtd) * (dc + Jt * at_)

    c = [eye(2) Jd'] * Et' * (ct + Mt*Et*[zeros(2,1); ad]) + J'*Psit'*c0r; % if c0r and c0p are 0 the second term is 0

    % TT = M * qdda + c
    % qdda_ = inv(M) * (TT-c)
    % T
    qdda = inv(M) * (T-c);
